simulink model "TestStructure"  (R2023b)
settings: Solver=FixedStepDiscrete  StartTime=0.0  StopTime=inf  FixedStep=SampleTime  RelTol=1e-3
InitFcn:
  | SampleTime = 0.001;
  | ButtonValue=0;
  | load("BusConfig.mat");
undefined symbols (not defined in the file): DiscIntNeverNeededParam
libraries: slrealtimeethercatlib x219, dspfdesign x28, dspstat3 x23, simulink x21, slpidlib x10, dspswit3 x8, commfilt2 x2, dspsigops x1
(part 7 of 8)

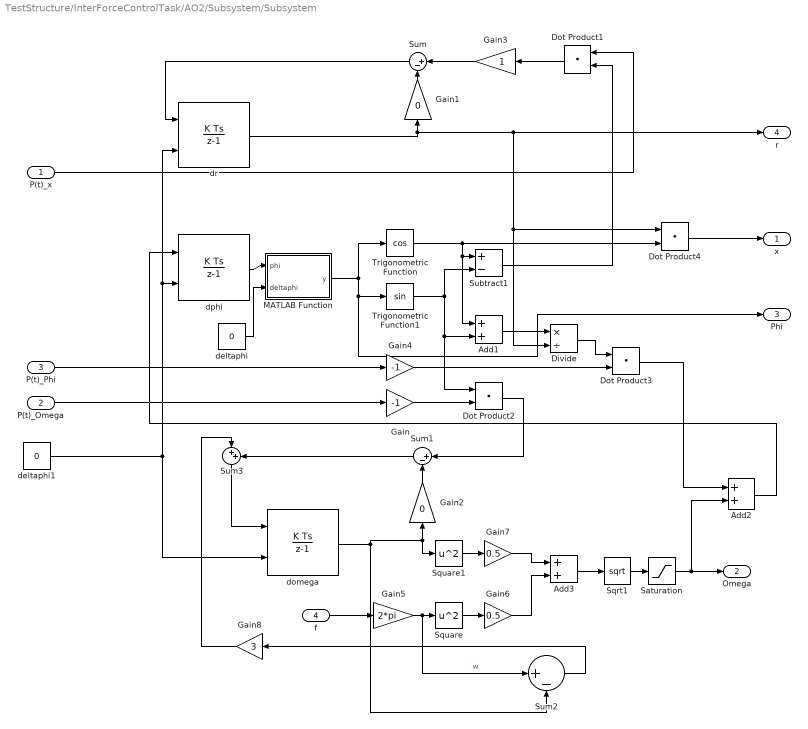
== system TestStructure/InterForceControlTask/AO2/Subsystem/Subsystem ==
  P(t)_x : Inport
  P(t)_Omega : Inport  Port=2
  P(t)_Phi : Inport  Port=3
  f : Inport  Port=4
  Add1 : Sum
  Add2 : Sum
  Add3 : Sum
  Divide : Product  Inputs=*/
  Dot Product{1..4} (4 alike) : DotProduct  OutDataTypeStr=Inherit: Inherit via internal rule
  Gain : Gain  Gain=-1
  Gain1 : Gain  Gain=0
  Gain2 : Gain  Gain=0
  Gain3 : Gain
  Gain4 : Gain  Gain=-1
  Gain5 : Gain  Gain=2*pi
  Gain6 : Gain  Gain=0.5
  Gain7 : Gain  Gain=0.5
  Gain8 : Gain  Gain=3
  MATLAB Function : MATLAB Function  TreatAsAtomicUnit=on
  Saturation : Saturate  UpperLimit=2*pi*1  LowerLimit=2*pi*0.15
  Sqrt1 : Sqrt
  Square : Math  Operator=square
  Square1 : Math  Operator=square
  Subtract1 : Sum  Inputs=+-
  Sum : Sum  Inputs=|+-
  Sum1 : Sum  Inputs=|+-
  Sum2 : Sum  Inputs=|+-
  Sum3 : Sum  Inputs=|++
  Trigonometric Function : Trigonometry  Operator=cos
  Trigonometric Function1 : Trigonometry
  deltaphi : Constant  Value=0
  deltaphi1 : Constant  Value=0
  domega : DiscreteIntegrator  ExternalReset=falling  InitialCondition=0.3*2*pi  SampleTime=-1  LimitOutput=on  UpperSaturationLimit=2*pi*0.9  LowerSaturationLimit=2*pi*0.15  ICPrevOutput=DiscIntNeverNeededParam  ICPrevScaledInput=DiscIntNeverNeededParam
  dphi : DiscreteIntegrator  ExternalReset=falling  InitialCondition=1  SampleTime=-1  ICPrevOutput=DiscIntNeverNeededParam  ICPrevScaledInput=DiscIntNeverNeededParam
  dr : DiscreteIntegrator  ExternalReset=falling  InitialCondition=1  SampleTime=-1  ICPrevOutput=DiscIntNeverNeededParam  ICPrevScaledInput=DiscIntNeverNeededParam
  x : Outport
  Omega : Outport  Port=2
  Phi : Outport  Port=3
  r : Outport  Port=4
  wires:
  Gain8/1 -> Sum3/1
  Sum3/1 -> domega/1
  Sum2/1 -> Gain8/1
  Gain6/1 -> Add3/2
  Gain7/1 -> Add3/1
  domega/1 -> Sum2/2, Gain2/1, Square1/1
  Square1/1 -> Gain7/1
  f/1 -> Gain5/1
  Square/1 -> Gain6/1
  Gain5/1 -> Square/1, Sum2/1  "w"
  Saturation/1 -> Omega/1, Add2/2
  Sqrt1/1 -> Saturation/1
  Add3/1 -> Sqrt1/1
  Gain4/1 -> Dot Product3/2
  P(t)_Omega/1 -> Gain/1
  P(t)_x/1 -> Dot Product1/1
  P(t)_Phi/1 -> Gain4/1
  Trigonometric Function/1 -> Dot Product4/2, Subtract1/1, Add1/1
  deltaphi1/1 -> domega/2, dphi/2, dr/2
  Gain3/1 -> Sum/1
  Sum/1 -> dr/1
  Gain2/1 -> Sum1/2
  Sum1/1 -> Sum3/2
  Gain1/1 -> Sum/2
  dr/1 -> r/1, Dot Product4/1, Divide/2, Gain1/1
  deltaphi/1 -> MATLAB Function/2(deltaphi)
  dphi/1 -> MATLAB Function/1(phi)
  Divide/1 -> Dot Product3/1
  Subtract1/1 -> Dot Product1/2
  Dot Product3/1 -> Add2/1
  Dot Product1/1 -> Gain3/1
  Trigonometric Function1/1 -> Dot Product2/1, Add1/2, Subtract1/2
  Dot Product4/1 -> x/1
  Gain/1 -> Dot Product2/2
  Dot Product2/1 -> Sum1/1
  MATLAB Function/1(y) -> Trigonometric Function1/1, Phi/1, Trigonometric Function/1
  Add1/1 -> Divide/1
  Add2/1 -> dphi/1

== system TestStructure/InterForceControlTask/AO2/Subsystem/Subsystem1 ==
  P(t)_x : Inport
  P(t)_Phi : Inport  Port=2
  Omega : Inport  Port=3
  Add1 : Sum
  Add2 : Sum
  Divide : Product  Inputs=*/
  Dot Product1 : DotProduct  OutDataTypeStr=Inherit: Inherit via internal rule
  Dot Product3 : DotProduct  OutDataTypeStr=Inherit: Inherit via internal rule
  Dot Product4 : DotProduct  OutDataTypeStr=Inherit: Inherit via internal rule
  Gain : Gain  Gain=2
  Gain1 : Gain  Gain=0
  Gain3 : Gain
  Gain4 : Gain  Gain=-1
  MATLAB Function : MATLAB Function  TreatAsAtomicUnit=on
  Subtract1 : Sum  Inputs=+-
  Sum : Sum  Inputs=|+-
  Trigonometric Function : Trigonometry  Operator=cos
  Trigonometric Function1 : Trigonometry
  deltaphi : Constant  Value=0
  deltaphi1 : Constant  Value=0
  dphi : DiscreteIntegrator  ExternalReset=falling  InitialCondition=1  SampleTime=-1  ICPrevOutput=DiscIntNeverNeededParam  ICPrevScaledInput=DiscIntNeverNeededParam
  dr : DiscreteIntegrator  ExternalReset=falling  InitialCondition=1  SampleTime=-1  ICPrevOutput=DiscIntNeverNeededParam  ICPrevScaledInput=DiscIntNeverNeededParam
  x : Outport
  Phi : Outport  Port=2
  r : Outport  Port=3
  wires:
  Gain/1 -> Add2/2
  Gain4/1 -> Dot Product3/2
  P(t)_x/1 -> Dot Product1/1
  P(t)_Phi/1 -> Gain4/1
  Trigonometric Function/1 -> Dot Product4/2, Subtract1/1, Add1/1
  deltaphi1/1 -> dphi/2, dr/2
  Gain3/1 -> Sum/1
  Sum/1 -> dr/1
  Gain1/1 -> Sum/2
  dr/1 -> Gain1/1, r/1, Dot Product4/1, Divide/2
  deltaphi/1 -> MATLAB Function/2(deltaphi)
  dphi/1 -> MATLAB Function/1(phi)
  Divide/1 -> Dot Product3/1
  Subtract1/1 -> Dot Product1/2
  Dot Product3/1 -> Add2/1
  Dot Product1/1 -> Gain3/1
  Omega/1 -> Gain/1
  Trigonometric Function1/1 -> Add1/2, Subtract1/2
  Dot Product4/1 -> x/1
  MATLAB Function/1(y) -> Trigonometric Function1/1, Phi/1, Trigonometric Function/1
  Add1/1 -> Divide/1
  Add2/1 -> dphi/1

== system TestStructure/InterForceControlTask/AO2/Subsystem/Subsystem2 ==
  note: 交替打腿 7.5 0.7
  T(t) : Inport
  X(t) : Inport  Port=2
  Reset : Inport  Port=3
  0.1 : Gain  Gain=12
  0.2 : Gain  Gain=60
  0.3 : Gain  Gain=10
  0.4 : Gain  Gain=4
  Abs : Abs  SaturateOnIntegerOverflow=off
  Abs1 : Abs  SaturateOnIntegerOverflow=off
  Add3 : Sum  Inputs=+-+
  Add4 : Sum  Inputs=+-+
  Discrete Derivative : simulink/Discrete/Discrete Derivative  gainval=1.0  ICPrevScaledInput=0.0  OutMin=[]  OutMax=[]  OutDataType=fixdt(1, 16)  OutScaling=2^-10  DoSatur=off
  Discrete Derivative1 : simulink/Discrete/Discrete Derivative  gainval=1.0  ICPrevScaledInput=0.0  OutMin=[]  OutMax=[]  OutDataType=fixdt(1, 16)  OutScaling=2^-10  DoSatur=off
  Discrete-Time Integrator3 : DiscreteIntegrator  ExternalReset=falling  InitialCondition=0.1  SampleTime=-1  ICPrevOutput=DiscIntNeverNeededParam  ICPrevScaledInput=DiscIntNeverNeededParam
  Discrete-Time Integrator4 : DiscreteIntegrator  ExternalReset=falling  InitialCondition=0.01  SampleTime=-1  ICPrevOutput=DiscIntNeverNeededParam  ICPrevScaledInput=DiscIntNeverNeededParam
  Dot Product{1..3,5..7,10} (7 alike) : DotProduct  OutDataTypeStr=Inherit: Inherit via internal rule
  Gain : Gain  Gain=10
  Gain1 : Gain  Gain=3
  Saturation : Saturate  UpperLimit=40  LowerLimit=0
  Saturation3 : Saturate  UpperLimit=40  LowerLimit=0
  Subtract2 : Sum
  Sum1 : Sum  Inputs=-+|
  Sum2 : Sum  Inputs=-+|
  amp1 : Gain
  amp2 : Gain
  eta_0 : Constant  Value=2
  eta_1 : Constant
  eta_2 : Constant  Value=20
  P(t)_x : Outport
  P(t)_Omega : Outport  Port=2
  P(t)_Phi : Outport  Port=3
  P : Outport  Port=4
  wires:
  Gain1/1 -> P(t)_Phi/1
  Gain/1 -> P(t)_Omega/1
  Dot Product3/1 -> P(t)_x/1  "P"
  Dot Product2/1 -> Gain1/1  "P"
  Subtract2/1 -> Dot Product1/2, Dot Product2/2, P/1, Dot Product3/2  "P"
  Dot Product5/1 -> Abs/1
  Discrete Derivative1/1 -> Sum2/2
  Discrete Derivative/1 -> Sum2/1
  Reset/1 -> Discrete-Time Integrator4/2, Discrete-Time Integrator3/2
  0.4/1 -> Add4/2
  0.3/1 -> Add3/2
  Saturation3/1 -> Subtract2/2, Dot Product7/2
  amp2/1 -> Dot Product5/1
  Saturation/1 -> Dot Product5/2, Subtract2/1
  Dot Product1/1 -> Gain/1  "P"
  Abs1/1 -> Dot Product6/2
  eta_0/1 -> Add3/1
  Dot Product6/1 -> 0.2/1  "eta"
  Abs/1 -> Dot Product10/2
  eta_1/1 -> Dot Product10/1, Dot Product6/1
  amp1/1 -> Dot Product1/1, Dot Product3/1, Dot Product2/1, Dot Product7/1  "eta"
  Sum2/1 -> amp2/1
  Sum1/1 -> amp1/1  "F"
  T(t)/1 -> Sum1/2, Discrete Derivative1/1
  Add3/1 -> Discrete-Time Integrator4/1
  X(t)/1 -> Discrete Derivative/1, Sum1/1
  eta_2/1 -> Add4/1
  Add4/1 -> Discrete-Time Integrator3/1
  0.1/1 -> Add3/3
  Discrete-Time Integrator4/1 -> Saturation/1, 0.3/1  "eta"
  Dot Product10/1 -> 0.1/1  "eta"
  Dot Product7/1 -> Abs1/1
  0.2/1 -> Add4/3
  Discrete-Time Integrator3/1 -> Saturation3/1, 0.4/1  "eta"

== system TestStructure/InterForceControlTask/AO2/Subsystem/Subsystem3 ==
  P(t)_x : Inport
  Omega : Inport  Port=2
  P(t)_Phi : Inport  Port=3
  Add1 : Sum
  Add2 : Sum
  Divide : Product  Inputs=*/
  Dot Product1 : DotProduct  OutDataTypeStr=Inherit: Inherit via internal rule
  Dot Product3 : DotProduct  OutDataTypeStr=Inherit: Inherit via internal rule
  Dot Product4 : DotProduct  OutDataTypeStr=Inherit: Inherit via internal rule
  Gain : Gain  Gain=3
  Gain1 : Gain  Gain=0
  Gain3 : Gain
  Gain4 : Gain  Gain=-1
  MATLAB Function : MATLAB Function  TreatAsAtomicUnit=on
  Subtract1 : Sum  Inputs=+-
  Sum : Sum  Inputs=|+-
  Trigonometric Function : Trigonometry  Operator=cos
  Trigonometric Function1 : Trigonometry
  d : Constant  Value=0
  deltaphi : Constant  Value=0
  dphi : DiscreteIntegrator  ExternalReset=falling  InitialCondition=1  SampleTime=-1  ICPrevOutput=DiscIntNeverNeededParam  ICPrevScaledInput=DiscIntNeverNeededParam
  dr : DiscreteIntegrator  ExternalReset=falling  InitialCondition=1  SampleTime=-1  ICPrevOutput=DiscIntNeverNeededParam  ICPrevScaledInput=DiscIntNeverNeededParam
  x : Outport
  Phi : Outport  Port=2
  r : Outport  Port=3
  wires:
  Gain/1 -> Add2/2
  Gain4/1 -> Dot Product3/2
  P(t)_x/1 -> Dot Product1/1
  P(t)_Phi/1 -> Gain4/1
  Trigonometric Function/1 -> Dot Product4/2, Subtract1/1, Add1/1
  d/1 -> dphi/2, dr/2
  Gain3/1 -> Sum/1
  Sum/1 -> dr/1
  Gain1/1 -> Sum/2
  dr/1 -> Gain1/1, r/1, Dot Product4/1, Divide/2
  deltaphi/1 -> MATLAB Function/2(deltaphi)
  dphi/1 -> MATLAB Function/1(phi)
  Divide/1 -> Dot Product3/1
  Subtract1/1 -> Dot Product1/2
  Dot Product3/1 -> Add2/1
  Dot Product1/1 -> Gain3/1
  Omega/1 -> Gain/1
  Trigonometric Function1/1 -> Add1/2, Subtract1/2
  Dot Product4/1 -> x/1
  MATLAB Function/1(y) -> Trigonometric Function1/1, Phi/1, Trigonometric Function/1
  Add1/1 -> Divide/1
  Add2/1 -> dphi/1

== system TestStructure/InterForceControlTask/AO2/Subsystem/Subsystem5 ==
  P(t)_x : Inport
  P(t)_Phi : Inport  Port=2
  Omega : Inport  Port=3
  Add1 : Sum
  Add2 : Sum
  Divide : Product  Inputs=*/
  Dot Product1 : DotProduct  OutDataTypeStr=Inherit: Inherit via internal rule
  Dot Product3 : DotProduct  OutDataTypeStr=Inherit: Inherit via internal rule
  Dot Product4 : DotProduct  OutDataTypeStr=Inherit: Inherit via internal rule
  Gain : Gain  Gain=4
  Gain1 : Gain  Gain=0
  Gain3 : Gain
  Gain4 : Gain  Gain=-1
  MATLAB Function : MATLAB Function  TreatAsAtomicUnit=on
  Subtract1 : Sum  Inputs=+-
  Sum : Sum  Inputs=|+-
  Trigonometric Function : Trigonometry  Operator=cos
  Trigonometric Function1 : Trigonometry
  deltaphi : Constant  Value=0
  deltaphi1 : Constant  Value=0
  dphi : DiscreteIntegrator  ExternalReset=falling  InitialCondition=1  SampleTime=-1  ICPrevOutput=DiscIntNeverNeededParam  ICPrevScaledInput=DiscIntNeverNeededParam
  dr : DiscreteIntegrator  ExternalReset=falling  InitialCondition=1  SampleTime=-1  ICPrevOutput=DiscIntNeverNeededParam  ICPrevScaledInput=DiscIntNeverNeededParam
  x : Outport
  Phi : Outport  Port=2
  r : Outport  Port=3
  wires:
  Gain/1 -> Add2/2
  Gain4/1 -> Dot Product3/2
  P(t)_x/1 -> Dot Product1/1
  P(t)_Phi/1 -> Gain4/1
  Trigonometric Function/1 -> Dot Product4/2, Subtract1/1, Add1/1
  deltaphi1/1 -> dphi/2, dr/2
  Gain3/1 -> Sum/1
  Sum/1 -> dr/1
  Gain1/1 -> Sum/2
  dr/1 -> Gain1/1, r/1, Dot Product4/1, Divide/2
  deltaphi/1 -> MATLAB Function/2(deltaphi)
  dphi/1 -> MATLAB Function/1(phi)
  Divide/1 -> Dot Product3/1
  Subtract1/1 -> Dot Product1/2
  Dot Product3/1 -> Add2/1
  Dot Product1/1 -> Gain3/1
  Omega/1 -> Gain/1
  Trigonometric Function1/1 -> Add1/2, Subtract1/2
  Dot Product4/1 -> x/1
  MATLAB Function/1(y) -> Trigonometric Function1/1, Phi/1, Trigonometric Function/1
  Add1/1 -> Divide/1
  Add2/1 -> dphi/1

== system TestStructure/InterForceControlTask/AO2/Subsystem1/Subsystem ==
  Peaks : Inport
  Constant3 : Constant
  Discrete-Time Integrator : DiscreteIntegrator  ExternalReset=rising  SampleTime=-1  ICPrevOutput=DiscIntNeverNeededParam  ICPrevScaledInput=DiscIntNeverNeededParam
  If : If  IfExpression=u1 == 1
  If Action Subsystem : Subsystem  TreatAsAtomicUnit=on
  If Action Subsystem1 : Subsystem  TreatAsAtomicUnit=on
  Memory : Memory
  Merge : Merge
  Triggered Subsystem : Subsystem  TreatAsAtomicUnit=on
  t-t_start : Outport
  wires:
  Memory/1 -> Triggered Subsystem/1(In1)
  Triggered Subsystem/1(t-t_start) -> t-t_start/1
  If Action Subsystem/1(Out1) -> Merge/1
  If Action Subsystem1/1(Out1) -> Merge/2
  Constant3/1 -> Discrete-Time Integrator/1
  If/1 -> If Action Subsystem/Action
  Merge/1 -> Triggered Subsystem/Trigger, Discrete-Time Integrator/2
  If/2 -> If Action Subsystem1/Action
  Peaks/1 -> If/1
  Discrete-Time Integrator/1 -> Memory/1

== system TestStructure/InterForceControlTask/AO2/Subsystem1/ZeroCrossFinder ==
  q : Inport
  Discrete Derivative : simulink/Discrete/Discrete Derivative  gainval=1.0  ICPrevScaledInput=0.0  OutMin=[]  OutMax=[]  OutDataType=fixdt(1, 16)  OutScaling=2^-10  DoSatur=off
  If : If
  If Action Subsystem : Subsystem  TreatAsAtomicUnit=on
  If Action Subsystem1 : Subsystem  TreatAsAtomicUnit=on
  Merge : Merge
  Moving Maximum : dspstat3/Moving Maximum  SpecifyWindowLength=on  WindowLength=3  SimulateUsing=Code generation
  Moving Minimum : dspstat3/Moving Minimum  SpecifyWindowLength=on  WindowLength=3  SimulateUsing=Code generation
  Sign : Signum
  Cross : Outport
  wires:
  Moving Maximum/1 -> If Action Subsystem1/2(WindowMax)
  Moving Minimum/1 -> If Action Subsystem/2(WindowMin)
  q/1 -> Moving Maximum/1, Discrete Derivative/1, If Action Subsystem/1(q), If Action Subsystem1/1(q), Moving Minimum/1
  If Action Subsystem1/1(Out1) -> Merge/2
  If Action Subsystem/1(Out1) -> Merge/1
  Merge/1 -> Cross/1
  If/2 -> If Action Subsystem1/Action
  If/1 -> If Action Subsystem/Action
  Sign/1 -> If/1
  Discrete Derivative/1 -> Sign/1

== system TestStructure/InterForceControlTask/AO3/PhaseCorrection/If Action Subsystem ==
  Action Port : ActionPort
  Constant : Constant
  Out1 : Outport
  wires:
  Constant/1 -> Out1/1

== system TestStructure/InterForceControlTask/AO3/PhaseCorrection/If Action Subsystem1 ==
  Action Port : ActionPort
  Constant : Constant  Value=0
  Out1 : Outport
  wires:
  Constant/1 -> Out1/1

== system TestStructure/InterForceControlTask/AO3/Select/If Action Subsystem ==
  Phi : Inport
  Phase0 : Inport  Port=2
  Action Port : ActionPort  InitializeStates=reset
  Counter1 : dspswit3/Counter  Direction=Up  CountEvent=Rising edge  CounterSize=8 bits  MaxCount=255  InitialCount=0  Output=Count  HitValue=32  ResetInput=off  SamplesPerFrame=1  Ts=1  CntDtype=double  HitDtype=Logical
  If : If
  If Action Subsystem : Subsystem  TreatAsAtomicUnit=on
  If Action Subsystem1 : Subsystem  TreatAsAtomicUnit=on
  Merge : Merge
  Merge1 : Merge
  Phi_Out : Outport
  Phase0Event : Outport  Port=2
  wires:
  Phase0/1 -> If Action Subsystem/2(Phase0), Counter1/1
  Phi/1 -> If Action Subsystem/1(Phi)
  Counter1/1 -> If/1
  Merge/1 -> Phi_Out/1
  If/1 -> If Action Subsystem/Action
  If Action Subsystem/1(Out1) -> Merge/1
  If/2 -> If Action Subsystem1/Action
  If Action Subsystem1/1(Out1) -> Merge/2
  Merge1/1 -> Phase0Event/1
  If Action Subsystem1/2(Out2) -> Merge1/2
  If Action Subsystem/2(Out2) -> Merge1/1

== system TestStructure/InterForceControlTask/AO3/Select/If Action Subsystem1 ==
  Action Port : ActionPort
  Constant : Constant  Value=0
  Constant1 : Constant  Value=0
  Out1 : Outport
  Out2 : Outport  Port=2
  wires:
  Constant1/1 -> Out2/1
  Constant/1 -> Out1/1

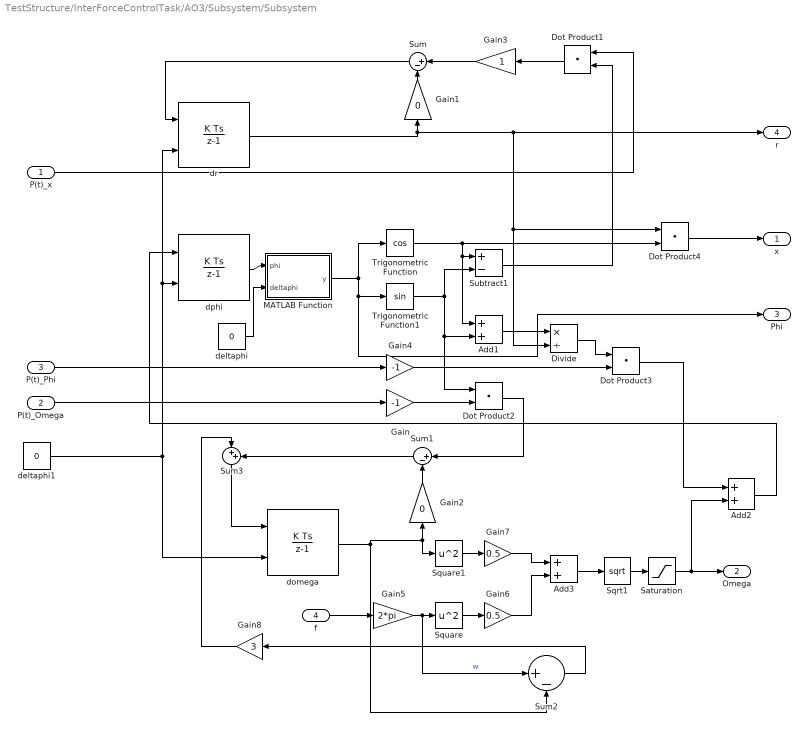
== system TestStructure/InterForceControlTask/AO3/Subsystem/Subsystem ==
  P(t)_x : Inport
  P(t)_Omega : Inport  Port=2
  P(t)_Phi : Inport  Port=3
  f : Inport  Port=4
  Add1 : Sum
  Add2 : Sum
  Add3 : Sum
  Divide : Product  Inputs=*/
  Dot Product{1..4} (4 alike) : DotProduct  OutDataTypeStr=Inherit: Inherit via internal rule
  Gain : Gain  Gain=-1
  Gain1 : Gain  Gain=0
  Gain2 : Gain  Gain=0
  Gain3 : Gain
  Gain4 : Gain  Gain=-1
  Gain5 : Gain  Gain=2*pi
  Gain6 : Gain  Gain=0.5
  Gain7 : Gain  Gain=0.5
  Gain8 : Gain  Gain=3
  MATLAB Function : MATLAB Function  TreatAsAtomicUnit=on
  Saturation : Saturate  UpperLimit=2*pi*1  LowerLimit=2*pi*0.15
  Sqrt1 : Sqrt
  Square : Math  Operator=square
  Square1 : Math  Operator=square
  Subtract1 : Sum  Inputs=+-
  Sum : Sum  Inputs=|+-
  Sum1 : Sum  Inputs=|+-
  Sum2 : Sum  Inputs=|+-
  Sum3 : Sum  Inputs=|++
  Trigonometric Function : Trigonometry  Operator=cos
  Trigonometric Function1 : Trigonometry
  deltaphi : Constant  Value=0
  deltaphi1 : Constant  Value=0
  domega : DiscreteIntegrator  ExternalReset=falling  InitialCondition=0.3*2*pi  SampleTime=-1  LimitOutput=on  UpperSaturationLimit=2*pi*0.9  LowerSaturationLimit=2*pi*0.15  ICPrevOutput=DiscIntNeverNeededParam  ICPrevScaledInput=DiscIntNeverNeededParam
  dphi : DiscreteIntegrator  ExternalReset=falling  InitialCondition=1  SampleTime=-1  ICPrevOutput=DiscIntNeverNeededParam  ICPrevScaledInput=DiscIntNeverNeededParam
  dr : DiscreteIntegrator  ExternalReset=falling  InitialCondition=1  SampleTime=-1  ICPrevOutput=DiscIntNeverNeededParam  ICPrevScaledInput=DiscIntNeverNeededParam
  x : Outport
  Omega : Outport  Port=2
  Phi : Outport  Port=3
  r : Outport  Port=4
  wires:
  Gain8/1 -> Sum3/1
  Sum3/1 -> domega/1
  Sum2/1 -> Gain8/1
  Gain6/1 -> Add3/2
  Gain7/1 -> Add3/1
  domega/1 -> Sum2/2, Gain2/1, Square1/1
  Square1/1 -> Gain7/1
  f/1 -> Gain5/1
  Square/1 -> Gain6/1
  Gain5/1 -> Square/1, Sum2/1  "w"
  Saturation/1 -> Omega/1, Add2/2
  Sqrt1/1 -> Saturation/1
  Add3/1 -> Sqrt1/1
  Gain4/1 -> Dot Product3/2
  P(t)_Omega/1 -> Gain/1
  P(t)_x/1 -> Dot Product1/1
  P(t)_Phi/1 -> Gain4/1
  Trigonometric Function/1 -> Dot Product4/2, Subtract1/1, Add1/1
  deltaphi1/1 -> domega/2, dphi/2, dr/2
  Gain3/1 -> Sum/1
  Sum/1 -> dr/1
  Gain2/1 -> Sum1/2
  Sum1/1 -> Sum3/2
  Gain1/1 -> Sum/2
  dr/1 -> r/1, Dot Product4/1, Divide/2, Gain1/1
  deltaphi/1 -> MATLAB Function/2(deltaphi)
  dphi/1 -> MATLAB Function/1(phi)
  Divide/1 -> Dot Product3/1
  Subtract1/1 -> Dot Product1/2
  Dot Product3/1 -> Add2/1
  Dot Product1/1 -> Gain3/1
  Trigonometric Function1/1 -> Dot Product2/1, Add1/2, Subtract1/2
  Dot Product4/1 -> x/1
  Gain/1 -> Dot Product2/2
  Dot Product2/1 -> Sum1/1
  MATLAB Function/1(y) -> Trigonometric Function1/1, Phi/1, Trigonometric Function/1
  Add1/1 -> Divide/1
  Add2/1 -> dphi/1

== system TestStructure/InterForceControlTask/AO3/Subsystem/Subsystem1 ==
  P(t)_x : Inport
  P(t)_Phi : Inport  Port=2
  Omega : Inport  Port=3
  Add1 : Sum
  Add2 : Sum
  Divide : Product  Inputs=*/
  Dot Product1 : DotProduct  OutDataTypeStr=Inherit: Inherit via internal rule
  Dot Product3 : DotProduct  OutDataTypeStr=Inherit: Inherit via internal rule
  Dot Product4 : DotProduct  OutDataTypeStr=Inherit: Inherit via internal rule
  Gain : Gain  Gain=2
  Gain1 : Gain  Gain=0
  Gain3 : Gain
  Gain4 : Gain  Gain=-1
  MATLAB Function : MATLAB Function  TreatAsAtomicUnit=on
  Subtract1 : Sum  Inputs=+-
  Sum : Sum  Inputs=|+-
  Trigonometric Function : Trigonometry  Operator=cos
  Trigonometric Function1 : Trigonometry
  deltaphi : Constant  Value=0
  deltaphi1 : Constant  Value=0
  dphi : DiscreteIntegrator  ExternalReset=falling  InitialCondition=1  SampleTime=-1  ICPrevOutput=DiscIntNeverNeededParam  ICPrevScaledInput=DiscIntNeverNeededParam
  dr : DiscreteIntegrator  ExternalReset=falling  InitialCondition=1  SampleTime=-1  ICPrevOutput=DiscIntNeverNeededParam  ICPrevScaledInput=DiscIntNeverNeededParam
  x : Outport
  Phi : Outport  Port=2
  r : Outport  Port=3
  wires:
  Gain/1 -> Add2/2
  Gain4/1 -> Dot Product3/2
  P(t)_x/1 -> Dot Product1/1
  P(t)_Phi/1 -> Gain4/1
  Trigonometric Function/1 -> Dot Product4/2, Subtract1/1, Add1/1
  deltaphi1/1 -> dphi/2, dr/2
  Gain3/1 -> Sum/1
  Sum/1 -> dr/1
  Gain1/1 -> Sum/2
  dr/1 -> Gain1/1, r/1, Dot Product4/1, Divide/2
  deltaphi/1 -> MATLAB Function/2(deltaphi)
  dphi/1 -> MATLAB Function/1(phi)
  Divide/1 -> Dot Product3/1
  Subtract1/1 -> Dot Product1/2
  Dot Product3/1 -> Add2/1
  Dot Product1/1 -> Gain3/1
  Omega/1 -> Gain/1
  Trigonometric Function1/1 -> Add1/2, Subtract1/2
  Dot Product4/1 -> x/1
  MATLAB Function/1(y) -> Trigonometric Function1/1, Phi/1, Trigonometric Function/1
  Add1/1 -> Divide/1
  Add2/1 -> dphi/1

== system TestStructure/InterForceControlTask/AO3/Subsystem/Subsystem2 ==
  note: 交替打腿 7.5 0.7
  T(t) : Inport
  X(t) : Inport  Port=2
  Reset : Inport  Port=3
  0.1 : Gain  Gain=12
  0.2 : Gain  Gain=60
  0.3 : Gain  Gain=10
  0.4 : Gain  Gain=4
  Abs : Abs  SaturateOnIntegerOverflow=off
  Abs1 : Abs  SaturateOnIntegerOverflow=off
  Add3 : Sum  Inputs=+-+
  Add4 : Sum  Inputs=+-+
  Discrete Derivative : simulink/Discrete/Discrete Derivative  gainval=1.0  ICPrevScaledInput=0.0  OutMin=[]  OutMax=[]  OutDataType=fixdt(1, 16)  OutScaling=2^-10  DoSatur=off
  Discrete Derivative1 : simulink/Discrete/Discrete Derivative  gainval=1.0  ICPrevScaledInput=0.0  OutMin=[]  OutMax=[]  OutDataType=fixdt(1, 16)  OutScaling=2^-10  DoSatur=off
  Discrete-Time Integrator3 : DiscreteIntegrator  ExternalReset=falling  InitialCondition=0.1  SampleTime=-1  ICPrevOutput=DiscIntNeverNeededParam  ICPrevScaledInput=DiscIntNeverNeededParam
  Discrete-Time Integrator4 : DiscreteIntegrator  ExternalReset=falling  InitialCondition=0.01  SampleTime=-1  ICPrevOutput=DiscIntNeverNeededParam  ICPrevScaledInput=DiscIntNeverNeededParam
  Dot Product{1..3,5..7,10} (7 alike) : DotProduct  OutDataTypeStr=Inherit: Inherit via internal rule
  Gain : Gain  Gain=10
  Gain1 : Gain  Gain=3
  Saturation : Saturate  UpperLimit=40  LowerLimit=0
  Saturation3 : Saturate  UpperLimit=40  LowerLimit=0
  Subtract2 : Sum
  Sum1 : Sum  Inputs=-+|
  Sum2 : Sum  Inputs=-+|
  amp1 : Gain
  amp2 : Gain
  eta_0 : Constant  Value=2
  eta_1 : Constant
  eta_2 : Constant  Value=20
  P(t)_x : Outport
  P(t)_Omega : Outport  Port=2
  P(t)_Phi : Outport  Port=3
  P : Outport  Port=4
  wires:
  Gain1/1 -> P(t)_Phi/1
  Gain/1 -> P(t)_Omega/1
  Dot Product3/1 -> P(t)_x/1  "P"
  Dot Product2/1 -> Gain1/1  "P"
  Subtract2/1 -> Dot Product1/2, Dot Product2/2, P/1, Dot Product3/2  "P"
  Dot Product5/1 -> Abs/1
  Discrete Derivative1/1 -> Sum2/2
  Discrete Derivative/1 -> Sum2/1
  Reset/1 -> Discrete-Time Integrator4/2, Discrete-Time Integrator3/2
  0.4/1 -> Add4/2
  0.3/1 -> Add3/2
  Saturation3/1 -> Subtract2/2, Dot Product7/2
  amp2/1 -> Dot Product5/1
  Saturation/1 -> Dot Product5/2, Subtract2/1
  Dot Product1/1 -> Gain/1  "P"
  Abs1/1 -> Dot Product6/2
  eta_0/1 -> Add3/1
  Dot Product6/1 -> 0.2/1  "eta"
  Abs/1 -> Dot Product10/2
  eta_1/1 -> Dot Product10/1, Dot Product6/1
  amp1/1 -> Dot Product1/1, Dot Product3/1, Dot Product2/1, Dot Product7/1  "eta"
  Sum2/1 -> amp2/1
  Sum1/1 -> amp1/1  "F"
  T(t)/1 -> Sum1/2, Discrete Derivative1/1
  Add3/1 -> Discrete-Time Integrator4/1
  X(t)/1 -> Discrete Derivative/1, Sum1/1
  eta_2/1 -> Add4/1
  Add4/1 -> Discrete-Time Integrator3/1
  0.1/1 -> Add3/3
  Discrete-Time Integrator4/1 -> Saturation/1, 0.3/1  "eta"
  Dot Product10/1 -> 0.1/1  "eta"
  Dot Product7/1 -> Abs1/1
  0.2/1 -> Add4/3
  Discrete-Time Integrator3/1 -> Saturation3/1, 0.4/1  "eta"

== system TestStructure/InterForceControlTask/AO3/Subsystem/Subsystem3 ==
  P(t)_x : Inport
  Omega : Inport  Port=2
  P(t)_Phi : Inport  Port=3
  Add1 : Sum
  Add2 : Sum
  Divide : Product  Inputs=*/
  Dot Product1 : DotProduct  OutDataTypeStr=Inherit: Inherit via internal rule
  Dot Product3 : DotProduct  OutDataTypeStr=Inherit: Inherit via internal rule
  Dot Product4 : DotProduct  OutDataTypeStr=Inherit: Inherit via internal rule
  Gain : Gain  Gain=3
  Gain1 : Gain  Gain=0
  Gain3 : Gain
  Gain4 : Gain  Gain=-1
  MATLAB Function : MATLAB Function  TreatAsAtomicUnit=on
  Subtract1 : Sum  Inputs=+-
  Sum : Sum  Inputs=|+-
  Trigonometric Function : Trigonometry  Operator=cos
  Trigonometric Function1 : Trigonometry
  d : Constant  Value=0
  deltaphi : Constant  Value=0
  dphi : DiscreteIntegrator  ExternalReset=falling  InitialCondition=1  SampleTime=-1  ICPrevOutput=DiscIntNeverNeededParam  ICPrevScaledInput=DiscIntNeverNeededParam
  dr : DiscreteIntegrator  ExternalReset=falling  InitialCondition=1  SampleTime=-1  ICPrevOutput=DiscIntNeverNeededParam  ICPrevScaledInput=DiscIntNeverNeededParam
  x : Outport
  Phi : Outport  Port=2
  r : Outport  Port=3
  wires:
  Gain/1 -> Add2/2
  Gain4/1 -> Dot Product3/2
  P(t)_x/1 -> Dot Product1/1
  P(t)_Phi/1 -> Gain4/1
  Trigonometric Function/1 -> Dot Product4/2, Subtract1/1, Add1/1
  d/1 -> dphi/2, dr/2
  Gain3/1 -> Sum/1
  Sum/1 -> dr/1
  Gain1/1 -> Sum/2
  dr/1 -> Gain1/1, r/1, Dot Product4/1, Divide/2
  deltaphi/1 -> MATLAB Function/2(deltaphi)
  dphi/1 -> MATLAB Function/1(phi)
  Divide/1 -> Dot Product3/1
  Subtract1/1 -> Dot Product1/2
  Dot Product3/1 -> Add2/1
  Dot Product1/1 -> Gain3/1
  Omega/1 -> Gain/1
  Trigonometric Function1/1 -> Add1/2, Subtract1/2
  Dot Product4/1 -> x/1
  MATLAB Function/1(y) -> Trigonometric Function1/1, Phi/1, Trigonometric Function/1
  Add1/1 -> Divide/1
  Add2/1 -> dphi/1

== system TestStructure/InterForceControlTask/AO3/Subsystem/Subsystem5 ==
  P(t)_x : Inport
  P(t)_Phi : Inport  Port=2
  Omega : Inport  Port=3
  Add1 : Sum
  Add2 : Sum
  Divide : Product  Inputs=*/
  Dot Product1 : DotProduct  OutDataTypeStr=Inherit: Inherit via internal rule
  Dot Product3 : DotProduct  OutDataTypeStr=Inherit: Inherit via internal rule
  Dot Product4 : DotProduct  OutDataTypeStr=Inherit: Inherit via internal rule
  Gain : Gain  Gain=4
  Gain1 : Gain  Gain=0
  Gain3 : Gain
  Gain4 : Gain  Gain=-1
  MATLAB Function : MATLAB Function  TreatAsAtomicUnit=on
  Subtract1 : Sum  Inputs=+-
  Sum : Sum  Inputs=|+-
  Trigonometric Function : Trigonometry  Operator=cos
  Trigonometric Function1 : Trigonometry
  deltaphi : Constant  Value=0
  deltaphi1 : Constant  Value=0
  dphi : DiscreteIntegrator  ExternalReset=falling  InitialCondition=1  SampleTime=-1  ICPrevOutput=DiscIntNeverNeededParam  ICPrevScaledInput=DiscIntNeverNeededParam
  dr : DiscreteIntegrator  ExternalReset=falling  InitialCondition=1  SampleTime=-1  ICPrevOutput=DiscIntNeverNeededParam  ICPrevScaledInput=DiscIntNeverNeededParam
  x : Outport
  Phi : Outport  Port=2
  r : Outport  Port=3
  wires:
  Gain/1 -> Add2/2
  Gain4/1 -> Dot Product3/2
  P(t)_x/1 -> Dot Product1/1
  P(t)_Phi/1 -> Gain4/1
  Trigonometric Function/1 -> Dot Product4/2, Subtract1/1, Add1/1
  deltaphi1/1 -> dphi/2, dr/2
  Gain3/1 -> Sum/1
  Sum/1 -> dr/1
  Gain1/1 -> Sum/2
  dr/1 -> Gain1/1, r/1, Dot Product4/1, Divide/2
  deltaphi/1 -> MATLAB Function/2(deltaphi)
  dphi/1 -> MATLAB Function/1(phi)
  Divide/1 -> Dot Product3/1
  Subtract1/1 -> Dot Product1/2
  Dot Product3/1 -> Add2/1
  Dot Product1/1 -> Gain3/1
  Omega/1 -> Gain/1
  Trigonometric Function1/1 -> Add1/2, Subtract1/2
  Dot Product4/1 -> x/1
  MATLAB Function/1(y) -> Trigonometric Function1/1, Phi/1, Trigonometric Function/1
  Add1/1 -> Divide/1
  Add2/1 -> dphi/1

== system TestStructure/InterForceControlTask/AO3/Subsystem1/If Action Subsystem ==
  Action Port : ActionPort
  Constant : Constant
  Out1 : Outport
  wires:
  Constant/1 -> Out1/1

== system TestStructure/InterForceControlTask/AO3/Subsystem1/If Action Subsystem1 ==
  Action Port : ActionPort
  Constant : Constant  Value=0
  Out1 : Outport
  wires:
  Constant/1 -> Out1/1

== system TestStructure/InterForceControlTask/AO3/Subsystem1/If Action Subsystem2 ==
  q : Inport
  WindowMin : Inport  Port=2
  Action Port : ActionPort
  Function-Call Subsystem : Subsystem  TreatAsAtomicUnit=on
  Function-Call Subsystem1 : Subsystem  TreatAsAtomicUnit=on
  If : If  NumInputs=2  IfExpression=(u1 == 1)&(u2 == -1)
  Merge : Merge
  Sign : Signum
  Sign1 : Signum
  Out1 : Outport
  wires:
  Sign1/1 -> If/2
  Sign/1 -> If/1
  WindowMin/1 -> Sign1/1
  Function-Call Subsystem1/1(Out1) -> Merge/2
  Function-Call Subsystem/1(Out1) -> Merge/1
  Merge/1 -> Out1/1
  If/2 -> Function-Call Subsystem1/Action
  If/1 -> Function-Call Subsystem/Action
  q/1 -> Sign/1

== system TestStructure/InterForceControlTask/AO3/Subsystem1/If Action Subsystem3 ==
  q : Inport
  WindowMax : Inport  Port=2
  Action Port : ActionPort
  Function-Call Subsystem : Subsystem  TreatAsAtomicUnit=on
  Function-Call Subsystem1 : Subsystem  TreatAsAtomicUnit=on
  If : If  NumInputs=2  IfExpression=(u1 == -1) & (u2 == 1)
  Merge : Merge
  Sign : Signum
  Sign1 : Signum
  Out1 : Outport
  wires:
  Sign1/1 -> If/2
  Sign/1 -> If/1
  Merge/1 -> Out1/1
  WindowMax/1 -> Sign1/1
  q/1 -> Sign/1
  If/2 -> Function-Call Subsystem1/Action
  Function-Call Subsystem1/1(Out1) -> Merge/2
  If/1 -> Function-Call Subsystem/Action
  Function-Call Subsystem/1(Out1) -> Merge/1

== system TestStructure/InterForceControlTask/AO3/Subsystem1/Triggered Subsystem ==
  In1 : Inport
  Trigger : TriggerPort  VariantControl=(inherit)
  t-t_start : Outport
  wires:
  In1/1 -> t-t_start/1

== system TestStructure/InterForceControlTask/TorqueController/Subsystem2/Function-Call Subsystem ==
  Action Port : ActionPort  ActionPortLabel=if((u1 > u2))
  Constant : Constant
  Out1 : Outport
  wires:
  Constant/1 -> Out1/1

== system TestStructure/InterForceControlTask/TorqueController/Subsystem2/Function-Call Subsystem1 ==
  Action Port : ActionPort  ActionPortLabel=else
  Constant : Constant  Value=0
  Out1 : Outport
  wires:
  Constant/1 -> Out1/1

== system TestStructure/InterForceControlTask/TorqueController/Subsystem2/Function-Call Subsystem2 ==
  Action Port : ActionPort  ActionPortLabel=elseif((u1< -u2))
  Constant : Constant  Value=-1
  Out1 : Outport
  wires:
  Constant/1 -> Out1/1

== system TestStructure/InterForceControlTask/TorqueController/Subsystem2/If Action Subsystem2 ==
  WindowMin : Inport
  threadhold : Inport  Port=2
  Action Port : ActionPort  ActionPortLabel=if((u1 > -0.02)&(u1<0.02))
  Constant : Constant
  Function-Call Subsystem : Subsystem  TreatAsAtomicUnit=on
  Function-Call Subsystem1 : Subsystem  TreatAsAtomicUnit=on
  Function-Call Subsystem2 : Subsystem  TreatAsAtomicUnit=on
  If : If  IfExpression=(u1 > 0.4)  ElseIfExpressions=(u1< -0.4)
  MATLAB Function1 : MATLAB Function  TreatAsAtomicUnit=on
  Merge : Merge  Inputs=3
  Out1 : Outport
  Out2 : Outport  Port=2
  y : Outport  Port=3
  wires:
  If/1 -> Function-Call Subsystem/Action
  Merge/1 -> Out1/1
  Function-Call Subsystem/1(Out1) -> Merge/1  "1"
  Function-Call Subsystem1/1(Out1) -> Merge/3  "0"
  WindowMin/1 -> MATLAB Function1/1(u)
  If/3 -> Function-Call Subsystem1/Action
  If/2 -> Function-Call Subsystem2/Action
  Function-Call Subsystem2/1(Out1) -> Merge/2  "-1"
  MATLAB Function1/1(y) -> y/1, If/1
  Constant/1 -> Out2/1
  threadhold/1 -> MATLAB Function1/2(threadhold)

== system TestStructure/InterForceControlTask/TorqueController/Subsystem2/If Action Subsystem3 ==
  Action Port : ActionPort  ActionPortLabel=else
  Constant : Constant  Value=0
  Constant1 : Constant  Value=0
  Out1 : Outport
  Out2 : Outport  Port=2
  wires:
  Constant/1 -> Out1/1
  Constant1/1 -> Out2/1

== system TestStructure/InterForceControlTask/TorqueController2/ZeroCrossFinder_Right/If Action Subsystem1 ==
  WindowMin : Inport
  Action Port : ActionPort
  Function-Call Subsystem : Subsystem  TreatAsAtomicUnit=on
  Function-Call Subsystem1 : Subsystem  TreatAsAtomicUnit=on
  Function-Call Subsystem2 : Subsystem  TreatAsAtomicUnit=on
  If : If  IfExpression=(u1 > 0.4)  ElseIfExpressions=(u1< -0.4)
  Merge : Merge  Inputs=3
  Out1 : Outport
  wires:
  Function-Call Subsystem2/1(Out1) -> Merge/2
  If/2 -> Function-Call Subsystem2/Action
  If/3 -> Function-Call Subsystem1/Action
  WindowMin/1 -> If/1
  Function-Call Subsystem1/1(Out1) -> Merge/3
  Function-Call Subsystem/1(Out1) -> Merge/1
  Merge/1 -> Out1/1
  If/1 -> Function-Call Subsystem/Action

== system TestStructure/InterForceControlTask/TorqueController2/ZeroCrossFinder_Right/If Action Subsystem4 ==
  Action Port : ActionPort
  Constant : Constant  Value=0
  Out1 : Outport
  wires:
  Constant/1 -> Out1/1

== system TestStructure/InterForceControlTask/AO/Select/If Action Subsystem/If Action Subsystem ==
  Phi : Inport
  Phase0 : Inport  Port=2
  Action Port : ActionPort  ActionPortLabel=if(u1 > 0)
  Out1 : Outport
  Out2 : Outport  Port=2
  wires:
  Phase0/1 -> Out2/1
  Phi/1 -> Out1/1

== system TestStructure/InterForceControlTask/AO/Select/If Action Subsystem/If Action Subsystem1 ==
  Action Port : ActionPort  ActionPortLabel=else
  Constant : Constant  Value=0
  Constant1 : Constant  Value=0
  Out1 : Outport
  Out2 : Outport  Port=2
  wires:
  Constant1/1 -> Out2/1
  Constant/1 -> Out1/1

== system TestStructure/InterForceControlTask/AO/Subsystem1/If Action Subsystem2/Function-Call Subsystem ==
  Action Port : ActionPort  ActionPortLabel=if((u1 > 0.4))
  Constant : Constant
  Out1 : Outport
  wires:
  Constant/1 -> Out1/1

== system TestStructure/InterForceControlTask/AO/Subsystem1/If Action Subsystem2/Function-Call Subsystem1 ==
  Action Port : ActionPort  ActionPortLabel=else
  Constant : Constant  Value=0
  Out1 : Outport
  wires:
  Constant/1 -> Out1/1

== system TestStructure/InterForceControlTask/AO/Subsystem1/If Action Subsystem2/Function-Call Subsystem2 ==
  Action Port : ActionPort  ActionPortLabel=elseif((u1< -0.4))
  Constant : Constant  Value=-1
  Out1 : Outport
  wires:
  Constant/1 -> Out1/1

== system TestStructure/InterForceControlTask/AO1/Select/If Action Subsystem/If Action Subsystem ==
  Phi : Inport
  Phase0 : Inport  Port=2
  Action Port : ActionPort
  Out1 : Outport
  Out2 : Outport  Port=2
  wires:
  Phase0/1 -> Out2/1
  Phi/1 -> Out1/1

== system TestStructure/InterForceControlTask/AO1/Select/If Action Subsystem/If Action Subsystem1 ==
  Action Port : ActionPort
  Constant : Constant  Value=0
  Constant1 : Constant  Value=0
  Out1 : Outport
  Out2 : Outport  Port=2
  wires:
  Constant1/1 -> Out2/1
  Constant/1 -> Out1/1

== system TestStructure/InterForceControlTask/AO1/Subsystem1/If Action Subsystem2/Function-Call Subsystem ==
  Action Port : ActionPort
  Constant : Constant
  Out1 : Outport
  wires:
  Constant/1 -> Out1/1

== system TestStructure/InterForceControlTask/AO1/Subsystem1/If Action Subsystem2/Function-Call Subsystem1 ==
  Action Port : ActionPort
  Constant : Constant  Value=0
  Out1 : Outport
  wires:
  Constant/1 -> Out1/1

== system TestStructure/InterForceControlTask/AO1/Subsystem1/If Action Subsystem2/Function-Call Subsystem2 ==
  Action Port : ActionPort
  Constant : Constant  Value=-1
  Out1 : Outport
  wires:
  Constant/1 -> Out1/1

== system TestStructure/InterForceControlTask/AO2/PhaseCorrection/Subsystem/If Action Subsystem ==
  Action Port : ActionPort
  Constant : Constant
  Out1 : Outport
  wires:
  Constant/1 -> Out1/1

== system TestStructure/InterForceControlTask/AO2/PhaseCorrection/Subsystem/If Action Subsystem1 ==
  Action Port : ActionPort
  Constant : Constant  Value=0
  Out1 : Outport
  wires:
  Constant/1 -> Out1/1

== system TestStructure/InterForceControlTask/AO2/PhaseCorrection/Subsystem1/If Action Subsystem ==
  Action Port : ActionPort
  Constant : Constant
  Out1 : Outport
  wires:
  Constant/1 -> Out1/1

== system TestStructure/InterForceControlTask/AO2/PhaseCorrection/Subsystem1/If Action Subsystem1 ==
  Action Port : ActionPort
  Constant : Constant  Value=0
  Out1 : Outport
  wires:
  Constant/1 -> Out1/1

== system TestStructure/InterForceControlTask/AO2/PhaseCorrection/Subsystem1/Triggered Subsystem ==
  Phi_GP(t) : Inport
  Trigger : TriggerPort  VariantControl=(inherit)
  Phi_GP(t_start) : Outport
  wires:
  Phi_GP(t)/1 -> Phi_GP(t_start)/1

== system TestStructure/InterForceControlTask/AO2/PhaseCorrection/Subsystem2/If Action Subsystem ==
  Phi_GP(t_start) : Inport
  Action Port : ActionPort
  Gain : Gain  Gain=-1
  Out1 : Outport
  wires:
  Gain/1 -> Out1/1
  Phi_GP(t_start)/1 -> Gain/1

== system TestStructure/InterForceControlTask/AO2/PhaseCorrection/Subsystem2/If Action Subsystem1 ==
  Phi_GP(t_start) : Inport
  Action Port : ActionPort
  Bias : Bias  Bias=1  SaturateOnIntegerOverflow=off
  Gain : Gain  Gain=-1
  Out1 : Outport
  wires:
  Bias/1 -> Out1/1
  Gain/1 -> Bias/1
  Phi_GP(t_start)/1 -> Gain/1

== system TestStructure/InterForceControlTask/AO2/PhaseCorrection/Subsystem3/If Action Subsystem ==
  Action Port : ActionPort
  Constant : Constant
  Out1 : Outport
  wires:
  Constant/1 -> Out1/1

== system TestStructure/InterForceControlTask/AO2/PhaseCorrection/Subsystem3/If Action Subsystem1 ==
  Action Port : ActionPort
  Constant : Constant  Value=0
  Out1 : Outport
  wires:
  Constant/1 -> Out1/1

== system TestStructure/InterForceControlTask/AO2/PhaseCorrection/Subsystem3/Triggered Subsystem ==
  Phi_GP(t) : Inport
  Trigger : TriggerPort  VariantControl=(inherit)
  Phi_GP(t_start) : Outport
  wires:
  Phi_GP(t)/1 -> Phi_GP(t_start)/1

== system TestStructure/InterForceControlTask/AO2/Select/If Action Subsystem/If Action Subsystem ==
  Phi : Inport
  Phase0 : Inport  Port=2
  Action Port : ActionPort
  Out1 : Outport
  Out2 : Outport  Port=2
  wires:
  Phase0/1 -> Out2/1
  Phi/1 -> Out1/1

== system TestStructure/InterForceControlTask/AO2/Select/If Action Subsystem/If Action Subsystem1 ==
  Action Port : ActionPort
  Constant : Constant  Value=0
  Constant1 : Constant  Value=0
  Out1 : Outport
  Out2 : Outport  Port=2
  wires:
  Constant1/1 -> Out2/1
  Constant/1 -> Out1/1

== system TestStructure/InterForceControlTask/AO2/Subsystem1/Subsystem/If Action Subsystem ==
  Action Port : ActionPort
  Constant : Constant
  Out1 : Outport
  wires:
  Constant/1 -> Out1/1

== system TestStructure/InterForceControlTask/AO2/Subsystem1/Subsystem/If Action Subsystem1 ==
  Action Port : ActionPort
  Constant : Constant  Value=0
  Out1 : Outport
  wires:
  Constant/1 -> Out1/1

== system TestStructure/InterForceControlTask/AO2/Subsystem1/Subsystem/Triggered Subsystem ==
  In1 : Inport
  Trigger : TriggerPort  VariantControl=(inherit)
  t-t_start : Outport
  wires:
  In1/1 -> t-t_start/1

== system TestStructure/InterForceControlTask/AO2/Subsystem1/ZeroCrossFinder/If Action Subsystem ==
  q : Inport
  WindowMin : Inport  Port=2
  Action Port : ActionPort
  Function-Call Subsystem : Subsystem  TreatAsAtomicUnit=on
  Function-Call Subsystem1 : Subsystem  TreatAsAtomicUnit=on
  If : If  NumInputs=2  IfExpression=(u1 == 1)&(u2 == -1)
  Merge : Merge
  Sign : Signum
  Sign1 : Signum
  Out1 : Outport
  wires:
  Sign1/1 -> If/2
  Sign/1 -> If/1
  WindowMin/1 -> Sign1/1
  Function-Call Subsystem1/1(Out1) -> Merge/2
  Function-Call Subsystem/1(Out1) -> Merge/1
  Merge/1 -> Out1/1
  If/2 -> Function-Call Subsystem1/Action
  If/1 -> Function-Call Subsystem/Action
  q/1 -> Sign/1

== system TestStructure/InterForceControlTask/AO2/Subsystem1/ZeroCrossFinder/If Action Subsystem1 ==
  q : Inport
  WindowMax : Inport  Port=2
  Action Port : ActionPort
  Function-Call Subsystem : Subsystem  TreatAsAtomicUnit=on
  Function-Call Subsystem1 : Subsystem  TreatAsAtomicUnit=on
  If : If  NumInputs=2  IfExpression=(u1 == -1) & (u2 == 1)
  Merge : Merge
  Sign : Signum
  Sign1 : Signum
  Out1 : Outport
  wires:
  Sign1/1 -> If/2
  Sign/1 -> If/1
  Merge/1 -> Out1/1
  WindowMax/1 -> Sign1/1
  q/1 -> Sign/1
  If/2 -> Function-Call Subsystem1/Action
  Function-Call Subsystem1/1(Out1) -> Merge/2
  If/1 -> Function-Call Subsystem/Action
  Function-Call Subsystem/1(Out1) -> Merge/1

== system TestStructure/InterForceControlTask/AO3/Select/If Action Subsystem/If Action Subsystem ==
  Phi : Inport
  Phase0 : Inport  Port=2
  Action Port : ActionPort
  Out1 : Outport
  Out2 : Outport  Port=2
  wires:
  Phase0/1 -> Out2/1
  Phi/1 -> Out1/1

== system TestStructure/InterForceControlTask/AO3/Select/If Action Subsystem/If Action Subsystem1 ==
  Action Port : ActionPort
  Constant : Constant  Value=0
  Constant1 : Constant  Value=0
  Out1 : Outport
  Out2 : Outport  Port=2
  wires:
  Constant1/1 -> Out2/1
  Constant/1 -> Out1/1

== system TestStructure/InterForceControlTask/AO3/Subsystem1/If Action Subsystem2/Function-Call Subsystem ==
  Action Port : ActionPort
  Constant : Constant
  Out1 : Outport
  wires:
  Constant/1 -> Out1/1

== system TestStructure/InterForceControlTask/AO3/Subsystem1/If Action Subsystem2/Function-Call Subsystem1 ==
  Action Port : ActionPort
  Constant : Constant  Value=0
  Out1 : Outport
  wires:
  Constant/1 -> Out1/1

== system TestStructure/InterForceControlTask/AO3/Subsystem1/If Action Subsystem3/Function-Call Subsystem ==
  Action Port : ActionPort
  Constant : Constant  Value=-1
  Out1 : Outport
  wires:
  Constant/1 -> Out1/1

== system TestStructure/InterForceControlTask/AO3/Subsystem1/If Action Subsystem3/Function-Call Subsystem1 ==
  Action Port : ActionPort
  Constant : Constant  Value=0
  Out1 : Outport
  wires:
  Constant/1 -> Out1/1

== system TestStructure/InterForceControlTask/TorqueController/Subsystem2/If Action Subsystem2/Function-Call Subsystem ==
  Action Port : ActionPort  ActionPortLabel=if((u1 > 0.4))
  Constant : Constant
  Out1 : Outport
  wires:
  Constant/1 -> Out1/1

== system TestStructure/InterForceControlTask/TorqueController/Subsystem2/If Action Subsystem2/Function-Call Subsystem1 ==
  Action Port : ActionPort  ActionPortLabel=else
  Constant : Constant  Value=0
  Out1 : Outport
  wires:
  Constant/1 -> Out1/1

== system TestStructure/InterForceControlTask/TorqueController/Subsystem2/If Action Subsystem2/Function-Call Subsystem2 ==
  Action Port : ActionPort  ActionPortLabel=elseif((u1< -0.4))
  Constant : Constant  Value=-1
  Out1 : Outport
  wires:
  Constant/1 -> Out1/1

== system TestStructure/InterForceControlTask/TorqueController2/ZeroCrossFinder_Right/If Action Subsystem1/Function-Call Subsystem ==
  Action Port : ActionPort
  Constant : Constant
  Out1 : Outport
  wires:
  Constant/1 -> Out1/1

== system TestStructure/InterForceControlTask/TorqueController2/ZeroCrossFinder_Right/If Action Subsystem1/Function-Call Subsystem1 ==
  Action Port : ActionPort
  Constant : Constant  Value=0
  Out1 : Outport
  wires:
  Constant/1 -> Out1/1

== system TestStructure/InterForceControlTask/TorqueController2/ZeroCrossFinder_Right/If Action Subsystem1/Function-Call Subsystem2 ==
  Action Port : ActionPort
  Constant : Constant  Value=-1
  Out1 : Outport
  wires:
  Constant/1 -> Out1/1

== system TestStructure/InterForceControlTask/AO2/Subsystem1/ZeroCrossFinder/If Action Subsystem/Function-Call Subsystem ==
  Action Port : ActionPort
  Constant : Constant
  Out1 : Outport
  wires:
  Constant/1 -> Out1/1

== system TestStructure/InterForceControlTask/AO2/Subsystem1/ZeroCrossFinder/If Action Subsystem/Function-Call Subsystem1 ==
  Action Port : ActionPort
  Constant : Constant  Value=0
  Out1 : Outport
  wires:
  Constant/1 -> Out1/1

== system TestStructure/InterForceControlTask/AO2/Subsystem1/ZeroCrossFinder/If Action Subsystem1/Function-Call Subsystem ==
  Action Port : ActionPort
  Constant : Constant  Value=-1
  Out1 : Outport
  wires:
  Constant/1 -> Out1/1

== system TestStructure/InterForceControlTask/AO2/Subsystem1/ZeroCrossFinder/If Action Subsystem1/Function-Call Subsystem1 ==
  Action Port : ActionPort
  Constant : Constant  Value=0
  Out1 : Outport
  wires:
  Constant/1 -> Out1/1

== matlab function TestStructure/InterForceControlTask/AO/PhaseCorrection/MATLAB Function ==
  data: t_t_start input; Omega output; u input; phi output; T_base_default input
function [Omega, phi] = fcn(t_t_start, u, T_base_default)
%#codegen
% Hold the data-derived default until three complete AO periods exist.
persistent T1 T2 T3 T_avg_held measured_count prev_t prev_u
if isempty(T1)
    default_T = sanitizePeriod(T_base_default);
    T1 = default_T;
    T2 = default_T;
    T3 = default_T;
    T_avg_held = default_T;
    measured_count = int32(0);
    prev_t = 0.0;
    prev_u = 0.0;
end

if u > 0.5 && prev_u <= 0.5
    current_T = prev_t;
    % if current_T > 0.5 && current_T < 4.0
        T3 = T2;
        T2 = T1;
        T1 = current_T;
        measured_count = measured_count + 1;
        if measured_count >= 3
            T_avg_held = (T1 + T2 + T3) / 3.0;
        end
    % end
end

prev_t = t_t_start;
prev_u = u;
if T_avg_held > 0.1
    Omega = 1.0 / T_avg_held;
else
    Omega = 0.0;
end
phi = min(max(t_t_start * Omega, 0.0), 1.0);
end

function T = sanitizePeriod(value)
T = double(value);
if ~isfinite(T) || T <= 0.5 || T >= 4.0
    T = 1.66;
end
end

== matlab function TestStructure/InterForceControlTask/AO/PhaseCorrection/MATLAB Function1 ==
  data: raw_peak input; valid_peak output; t input
function valid_peak = Gait_Stabilizer(raw_peak, t)
    % raw_peak: 前端传来的完美瞬时脉冲
    % t: 仿真时间
    
    % 上次踩下的时间、上一步花了多久、当前是否稳定
    persistent last_peak_t T_prev is_stable
    
    if isempty(last_peak_t)
        last_peak_t = -10.0;
        T_prev = 0;
        is_stable = 0; % 默认：未稳定，冷眼旁观
    end
    
    valid_peak = 0; % 默认不输出
    
    % 突然停下来超过 2.5 秒没走
    % 系统立刻判定“失去稳态”，把大门关上，等你重新找回节奏
    if (t - last_peak_t) > 2.5
        is_stable = 0; 
    end
    
    % 当一个完美的物理脉冲到来时：
    if raw_peak > 0.5 
        
        % 算一下这一步花了多久
        T_curr = t - last_peak_t;
        
        % 过滤掉极度不合理的跨步（比如小于0.6秒的纯噪点，或大于2.5秒的停顿）
        if T_curr > 0.6 && T_curr < 2.5
            
            % 如果这一步的时间，跟上一步的时间，误差小于 0.2 秒
            if abs(T_curr - T_prev) < 0.2
                is_stable = 1; 
            else
                is_stable = 0; 
            end
            
            % 更新记忆，留给下一步对比
            T_prev = T_curr; 
        end
        
        if is_stable == 1
            valid_peak = 1;
        end
        
        last_peak_t = t; % 无论稳不稳定，都要记录这次物理脉冲发生的时间
    end
end

== matlab function TestStructure/InterForceControlTask/AO/PhaseCorrection/MATLAB Function2 ==
  data: valid_peak input; total_steps output
function total_steps = Step_Counter(valid_peak)
    % 只需记住当前的累计步数，和上次脉冲的状态（用来抓上升沿）
    persistent count prev_peak
    
    if isempty(count)
        count = 0;       % 开机步数为 0
        prev_peak = 0;
    end
    
    % 只有在完美脉冲抬头的瞬间，步数才 +1
    if valid_peak > 0.5 && prev_peak <= 0.5
        count = count + 1;
    end
    
    % 更新记忆，输出当前总步数
    prev_peak = valid_peak;
    total_steps = count;
end

== matlab function TestStructure/InterForceControlTask/AO/Select/MATLAB Function1 ==
  data: u input; y output
function y = fcn(u)
    y = (3/(1+exp(-40*(u+(1/10))))-3)+(3/(1+exp(-40*(u-(1/10)))));
end

== matlab function TestStructure/InterForceControlTask/AO/Subsystem1/Buffer Function ==
  data: u input; y output
function y = Buffer(u)
%#codegen
persistent buf

if isempty(buf)
    buf = zeros(30,1);
end

buf(1:29) = buf(2:30);
buf(30) = u;

y = buf;

== matlab function TestStructure/InterForceControlTask/DMP/MATLAB Function3 ==
  data: DataIn input; qWindowed output; Cross input; WinLen output; Enable output
function [qWindowed,WinLen,Enable] = SlidingWindowfcn(DataIn,Cross)
    persistent SlidingWindow;
    persistent OutputWindow;
    persistent SlidingWindowLength;
    persistent CrossCnt;
    persistent CrossPrevious;
    persistent win_1;
    persistent win_2;

    % base parameter
    winlen = 5000;
    interval = 10;

    % init
    if isempty(SlidingWindow)
        SlidingWindow = zeros(winlen,1);
        OutputWindow = zeros(winlen,1);
        SlidingWindowLength = 0;
        CrossCnt = 0;
        CrossPrevious = 0;
        win_1 = 0;
        win_2 = 0;
    end

    % sliding window
    if SlidingWindowLength == winlen
        SlidingWindow(1:winlen-1) = SlidingWindow(2:winlen);
        SlidingWindow(SlidingWindowLength) = DataIn;
        SlidingWindowLength = winlen;
        win_1 = win_1-1;
        win_2 = win_2-1;
        if(win_1<0)
            win_1 = 0;
        end
        if(win_2<0)
            win_2 = 0;
        end
        if (CrossPrevious == 0 && Cross == 1)
            if (CrossCnt==0)
                win_1 = SlidingWindowLength;
                CrossCnt = 1;
            else
                win_2 = SlidingWindowLength;
                CrossCnt = 0;
            end
        end
    else
        SlidingWindow(SlidingWindowLength+1) = DataIn;
        SlidingWindowLength = SlidingWindowLength + 1;
        if (CrossPrevious == 0 && Cross == 1)
            if (CrossCnt==0)
                win_1 = SlidingWindowLength;
                CrossCnt = 1;
            else
                win_2 = SlidingWindowLength;
                CrossCnt = 0;
            end
        end
    end
    CrossPrevious = Cross;

    WinLen = 0;
    % Trigger logic
    if (win_1~=0)&&(win_2~=0)
        if(win_1 > win_2)   
            WinLen = length(SlidingWindow(win_2:interval:win_1));
            OutputWindow(1:WinLen) = SlidingWindow(win_2:interval:win_1);
        elseif(win_1 < win_2)
            WinLen = length(SlidingWindow(win_1:interval:win_2));
            OutputWindow(1:WinLen) = SlidingWindow(win_1:interval:win_2);
        end
        Enable = 1;
        qWindowed = OutputWindow;
    else
        Enable = 0;
        WinLen = 0;
        qWindowed = zeros(winlen,1);
    end
end
